simulink model "Linearcontinious"  (R2018a)
settings: Solver=VariableStepAuto  StartTime=0.0  StopTime=2  RelTol=1e-3
values from neighbouring files (symbols this model uses):
  Bplus = 1    [Linearization&MDPP.m]
  pole1 = double(poles(2))    [Linearization&MDPP.m]
  pole2 = double(poles(3))    [Linearization&MDPP.m]
  Rprimedio = [1 rdio0]    [Linearization&MDPP.m]
  Sdio = [Sdio1 Sdio0]    [Linearization&MDPP.m]
  ttp = (Bmprimevec*A0)    [Linearization&MDPP.m]
undefined symbols (not defined in the file or in its folder): b
settings Model: Creator=Hirsa  LastModifiedBy=Hirsa

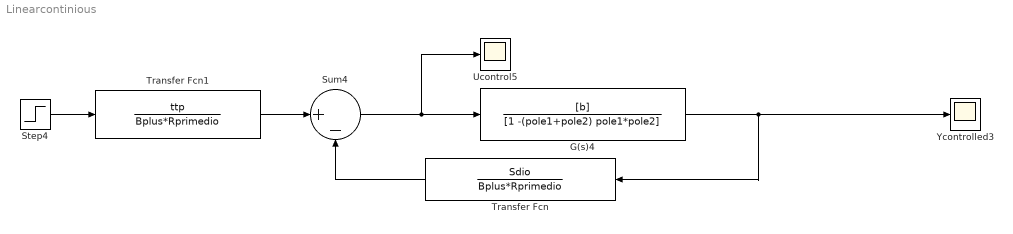
== system Linearcontinious ==
  G(s)4 : TransferFcn  Numerator=[b]  Denominator=[1 -(pole1+pole2) pole1*pole2]
  Step4 : Step
  Sum4 : Sum  Inputs=|+-
  Transfer Fcn : TransferFcn  Numerator=Sdio  Denominator=Bplus*Rprimedio
  Transfer Fcn1 : TransferFcn  Numerator=ttp  Denominator=Bplus*Rprimedio
  Ucontrol5 : Scope
  Ycontrolled3 : Scope
  wires:
  Sum4/1 -> Ucontrol5/1, G(s)4/1
  Step4/1 -> Transfer Fcn1/1
  G(s)4/1 -> Transfer Fcn/1, Ycontrolled3/1
  Transfer Fcn1/1 -> Sum4/1
  Transfer Fcn/1 -> Sum4/2
